simulink model "EX1_PID_pendulum_down"  (R2023b)
settings: Solver=FixedStepDiscrete  StartTime=0.0  StopTime=Inf  FixedStep=Ts  RelTol=1e-3  EnableMultiTasking=on
model workspace (MATLAB code in the model file):
  | % Processor Frequency
  | CPU_frequency = 90e6; %(Hz)
  | 
  | % PWM Settings
  | PWM_frequency = 15e3; %(Hz)
  | PWM_CounterPeriod = CPU_frequency/PWM_frequency/2; %(PWM timer counts)
  | 
  | % Switching frequency
  | fsw = PWM_frequency;
  | 
  | % Integration time (solver)
  | Ts = 1e-4;
  | 
  | % Encoder settings
  | fw = 400; % encoder sampling frequency
  | Tw = 1/fw; % encoder sampling time
values from neighbouring files (symbols this model uses):
  CALIBRATION_TIME = 50    [EX1_init.m]
  K_e = Distance / Encoder_Counts    (= 0.000124665903016)    [EX1_init.m]
  Kd = 0.2    [EX1_init.m]
  Ki = 0    [EX1_init.m]
  Kp = 10    [EX1_init.m]
  x_ref = 0    [EX1_init.m]
undefined symbols (not defined in the file or in its folder): DiscIntNeverNeededParam, Down, GPTRIP1SEL, GPTRIP2SEL, TZ1, TZ2, Up
libraries: c2802xlib x5, dspfdesign x2, simulink x2, c2806xlib x2, dspstat3 x2, c280xlib x1, eeGeneralControl x1, dspsigops x1
settings Model: ExtModeTrigDuration=8  Creator=The MathWorks, Inc.  LastModifiedBy=98912
settings SolverCC: AlgebraicLoopSolver=TrustRegion  AutoInsertRateTranBlk=on
settings OptimizationCC: DefaultUnderspecifiedDataType=single  EnhancedBackFolding=on  PassReuseOutputArgsAs=Individual arguments  MaxStackSize=1024  OptimizeBlockOrder=speed  DifferentSizesBufferReuse=on  OptimizationCustomize=off  DenormalBehavior=FlushToZero  EfficientTunableParamExpr=on
settings DebuggingCC: ParameterTunabilityLossMsg=error  UnconnectedInputMsg=warning  UnconnectedOutputMsg=warning  UnconnectedLineMsg=warning  SubsystemReferenceDiagnosticForUnitTest=warning
settings HardwareCC: ProdBitPerChar=16  ProdBitPerInt=16  ProdBitPerPointer=32  ProdBitPerSizeT=32  ProdBitPerPtrDiffT=32  ProdLargestAtomicInteger=Integer  ProdLargestAtomicFloat=None  ProdWordSize=16  ProdLongLongMode=on  ProdHWDeviceType=Texas Instruments->C2000
settings ModelReferenceCC: EnableRefExpFcnMdlSchedulingChecks=on
settings SFSimCC: MATLABDynamicMemAlloc=off
settings RTWCC: Description=Embedded Coder  SystemTargetFile=ert.tlc  HardwareBoard=TI Piccolo F28069M LaunchPad  TemplateMakefile=ert_default_tmf  GenerateReport=on  Toolchain=Texas Instruments Code Composer Studio (C2000)  DLArmComputeVersion=19.05
settings CodeAppCC: ForceParamTrailComments=on  IgnoreCustomStorageClasses=off  OperatorAnnotations=on  SimulinkDataObjDesc=on  SFDataObjDesc=on  InsertBlockDesc=on
settings ERTTargetCC: CodeReplacementLibrary=TI C28x  ExtModeStaticAllocSize=2000
settings SettingsController: UseSoCProfilerForTargets=0

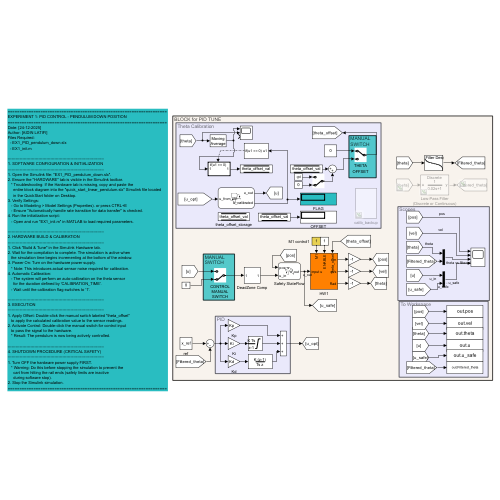
[thumbnail: Simulink's stored preview of the top-level diagram]
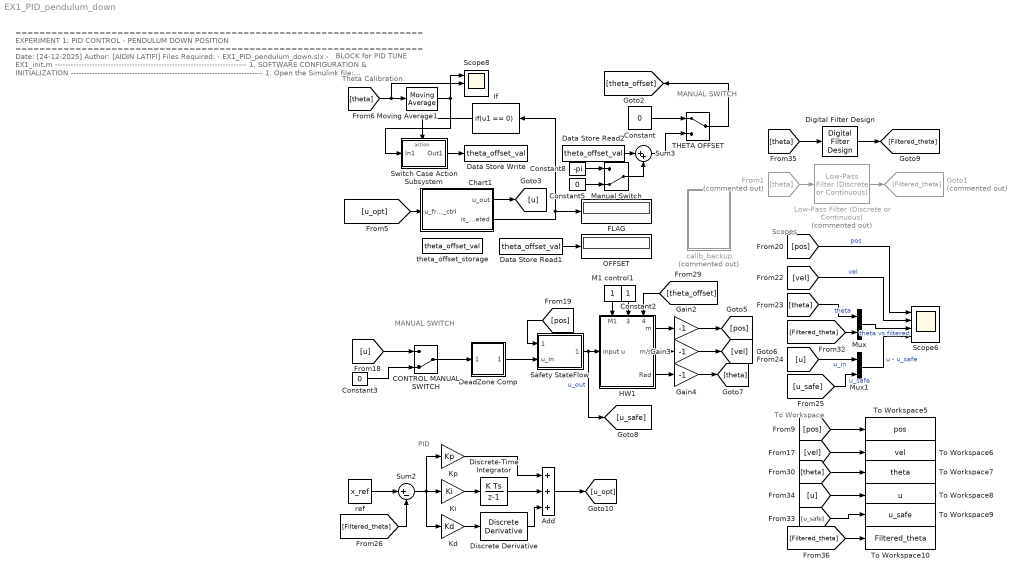
== system EX1_PID_pendulum_down ==
  note: MANUAL
      | SWITCH
  note: ====================================================================
      | EXPERIMENT 1: PID CONTROL - PENDULUM DOWN POSITION
      | ====================================================================
      | Date: [24-12-2025]
      | Author: [AIDIN LATIFI]
      | Files Required:
      |   - EX1_PID_pendulum_down.slx
      |   - EX1_init.m
      |
      | ------------------------------------------------------------------------
      | 1. SOFTWARE CONFIGURATION & INITIALIZATION
      | ------------------------------------------------------------------------
      | 1. Open the Simulink file: "EX1_PID_pendulum_down.slx".
      | 2. Ensure the "HARDWARE" tab is visible in the Simulink toolbar.
      |    * Troubleshooting: If the Hardware tab is missing, copy and paste the
      |      entire block diagram into the "quick_start_linear_pendulum.slx" Simulink file located
      |      in the QuickStart folder on Desktop.
      | 3. Verify Settings:
      |    - Go to Modeling > Model Settings (Properties). or press CTRL+E
      |    - Ensure "Automatically handle rate transition for data transfer" is checked.
      | 4. Run the initialization script:
      |    - Open and run "EX1_init.m" in MATLAB to load required parameters.
      |
      | ------------------------------------------------------------------------
      | 2. HARDWARE BUILD & CALIBRATION
      | ------------------------------------------------------------------------
      | 1. Click "Build & Tune" in the Simulink Hardware tab.
      | 2. Wait for the compilation to complete. The simulation is active when
      |    the simulation time begins incrementing at the bottom of the window.
      | 3. Power On: Turn on the hardware power supply.
      |    * Note: This introduces actual sensor noise required for calibration.
      | 4. Automatic Calibration:
      |    - The system will perform an auto-calibration on the theta sensor
      |      for the duration defined by 'CALIBRATION_TIME'.
      |    - Wait until the calibration flag switches to '1'.
      |
      | ------------------------------------------------------------------------
      | 3. EXECUTION
      | ------------------------------------------------------------------------
      | 1. Apply Offset: Double-click the manual switch labeled "theta_offset"
      |    to apply the calculated calibration value to the sensor readings.
      | 2. Activate Control: Double-click the manual switch for control input
      |    to pass the signal to the hardware.
      |    * Result: The pendulum is now being actively controlled.
      |
      | ------------------------------------------------------------------------
      | 4. SHUTDOWN PROCEDURE (CRITICAL SAFETY)
      | ------------------------------------------------------------------------
      | 1. Turn OFF the hardware power supply FIRST.
      |    * Warning: Do this before stopping the simulation to prevent the
      |      cart from hitting the rail ends (safety limits are inactive
      |      during software stop).
      | 2. Stop the Simulink simulation.
      | ====================================================================
  note: Theta Calibration
  note: To Workspace
  note: BLOCK for PID TUNE
  note: Scopes
  note: PID
  note: MANUAL
      | SWITCH
  Add : Sum  Inputs=+++
  CONTROL MANUAL SWITCH : ManualSwitch  CurrentSetting=0
  Chart1 : Stateflow chart  TreatAsAtomicUnit=on
  Constant : Constant  Value=0  SampleTime=Ts
  Constant2 : Constant
  Constant3 : Constant  Value=0  SampleTime=-1
  Constant5 : Constant  Value=0  SampleTime=Ts
  Constant8 : Constant  Value=-pi  SampleTime=Ts
  Data Store Read1 : DataStoreRead  DataStoreName=theta_offset_val  IndexOptions=Index vector (dialog)  Indices=1  OutputSizes=1
  Data Store Read2 : DataStoreRead  DataStoreName=theta_offset_val  IndexOptions=Index vector (dialog)  Indices=1  OutputSizes=1
  Data Store Write : DataStoreWrite  DataStoreName=theta_offset_val  IndexOptions=Index vector (dialog)  Indices=1  OutputSizes=1
  DeadZone Comp : Subsystem
  Digital Filter Design : dspfdesign/Digital Filter Design  mwdsp_browser_bugfix_var=off
  Discrete Derivative : simulink/Discrete/Discrete Derivative  gainval=1.0  ICPrevScaledInput=0.0  OutMin=[]  OutMax=[]  OutDataType=fixdt(1, 16)  OutScaling=2^-10  DoSatur=off
  Discrete-Time Integrator : DiscreteIntegrator  SampleTime=-1  LimitOutput=on  UpperSaturationLimit=2  LowerSaturationLimit=-2  ICPrevOutput=DiscIntNeverNeededParam  ICPrevScaledInput=DiscIntNeverNeededParam
  FLAG : Display
  From1 : From  Commented=on  GotoTag=theta
  Gain2 : Gain  Gain=-1
  Gain3 : Gain  Gain=-1
  Gain4 : Gain  Gain=-1
  Goto1 : Goto  Commented=on  GotoTag=Filtered_theta
  HW1 : Subsystem
      settings: PortSchema="{\"entries\":[{\"content\":{\"sides\":[{\"content\":{\"connectorIds\":[\"In1\"]},\"type\":\"ConnectorPlacement.EquallySpacedRectSide\",\"uuid\":\"e9898c75-a6e7-4646-b73a-b35b1fbe5adf\"},{\"content\":{\"connectorIds\":[\"Out1\",\"Out2\",\"Out3\"],\"side\":\"RIGHT\"},\"type\":\"ConnectorPlacement.EquallySpacedRectSide\",\"uuid\":\"085d2ccc-0e1f-4b16-8ec9-c70e62f660a1\"},{\"content\":{\"connectorIds\":[\"In2\",\"In3\",\"In4\"],\"side\":\"TOP\"},\"type\":\"ConnectorPlacement.EquallySpacedRectSide\",\"uuid\":\"51882789-74c2-4a7a-a001-ddaf25b9b479\"}]},\"type\":\"ConnectorPlacement.EquallySpacedConnector\",\"uuid\":\"373898fa-4a42-48b4-8ce1-77edd11dc4d5\"}],\"packageUris\":[\"http://schema.mathworks.com/mf0/Connector/R2020b\"],\"version\":\"1.0\"}"
  If : If  IfExpression=u1 == 0  ShowElse=off
  Kd : Gain  Gain=Kd
  Ki : Gain  Gain=Ki
  Kp : Gain  Gain=Kp
  Low-Pass Filter (Discrete or Continuous) : eeGeneralControl/Low-Pass Filter (Discrete or Continuous)  Commented=on  K=1  T=0.02  B=inf  A=-inf  init_option=Inherited from block input  x0=0  Ts=-1
  M1 control1 : Constant
  Manual Switch : ManualSwitch  CurrentSetting=0
  Moving Average1 : dspstat3/Moving Average  Method=Sliding window  ForgettingFactorPort=off  SpecifyWindowLength=off  WindowLength=200  OverlapLength=5  AllowArbitraryInputLength=off  ForgettingFactor=0.9  SimulateUsing=Interpreted execution
  Mux : Mux  Inputs=2
  Mux1 : Mux  Inputs=2
  OFFSET : Display
  Safety StateFlow : Stateflow chart  TreatAsAtomicUnit=on
  Scope6 : Scope  NumInputPorts=4
  Scope8 : Scope  NumInputPorts=3
  Sum2 : Sum  Inputs=|+-
  Sum3 : Sum  Inputs=|++
  Switch Case Action Subsystem : Subsystem  TreatAsAtomicUnit=on
  THETA OFFSET : ManualSwitch
  To Workspace10 : ToWorkspace  VariableName=Filtered_theta  SaveFormat=Timeseries  SampleTime=-1
  To Workspace5 : ToWorkspace  VariableName=pos  SaveFormat=Timeseries  SampleTime=-1
  To Workspace6 : ToWorkspace  VariableName=vel  SaveFormat=Timeseries  SampleTime=-1
  To Workspace7 : ToWorkspace  VariableName=theta  SaveFormat=Timeseries  SampleTime=-1
  To Workspace8 : ToWorkspace  VariableName=u  SaveFormat=Timeseries  SampleTime=-1
  To Workspace9 : ToWorkspace  VariableName=u_safe  SaveFormat=Timeseries  SampleTime=-1
  calib_backup : Subsystem  Commented=on
  ref : Constant  Value=x_ref  SampleTime=-1
  theta_offset_storage : DataStoreMemory  DataStoreName=theta_offset_val  WriteAfterWriteMsg=warning  ShowAdditionalParam=off
  wires:
  [u] -> CONTROL MANUAL SWITCH/1
  [u_safe] -> Mux1/2  "u_safe"
  [vel] -> To Workspace6/1
  Constant/1 -> THETA OFFSET/1
  [pos] -> Scope6/1  "pos"
  Add/1 -> [u_opt]
  Digital Filter Design/1 -> [Filtered_theta]
  [theta_offset] -> HW1/4(Theta_offset)
  Switch Case Action Subsystem/1(Out1) -> Data Store Write/1
  From1/1 -> Low-Pass Filter (Discrete or Continuous)/1
  Safety StateFlow/1(u_out) -> [u_safe], HW1/1(input u)  "u_out"
  Chart1/2(is_calibrated) -> FLAG/1, If/1
  THETA OFFSET/1 -> [theta_offset]
  Ki/1 -> Discrete-Time Integrator/1
  Sum3/1 -> THETA OFFSET/2
  [theta] -> Mux/1  "theta"
  Moving Average1/1 -> Switch Case Action Subsystem/1(In1), Scope8/1
  Data Store Read2/1 -> Sum3/1
  HW1/3(Rad) -> Gain4/1
  Manual Switch/1 -> Sum3/2
  Kd/1 -> Discrete Derivative/1
  Mux1/1 -> Scope6/4  "u - u_safe"
  [theta] -> Scope8/2, Moving Average1/1
  [u_opt] -> Chart1/1(u_from_ctrl)
  Chart1/1(u_out) -> [u]
  Mux/1 -> Scope6/3  "theta vs filtered"
  [Filtered_theta] -> To Workspace10/1
  HW1/2(m/s) -> Gain3/1
  [u] -> Mux1/1  "u_in"
  [pos] -> Safety StateFlow/1(pos_s)
  M1 control1/1 -> HW1/2(M1)
  Constant3/1 -> CONTROL MANUAL SWITCH/2
  Data Store Read1/1 -> OFFSET/1
  If/1 -> Switch Case Action Subsystem/Action
  [Filtered_theta] -> Mux/2
  ref/1 -> Sum2/1
  CONTROL MANUAL SWITCH/1 -> DeadZone Comp/1(In1)
  Constant2/1 -> HW1/3(ENABLE)
  Discrete Derivative/1 -> Add/3
  Constant5/1 -> Manual Switch/2
  Discrete-Time Integrator/1 -> Add/2
  Gain3/1 -> [vel]
  [u] -> To Workspace8/1
  [Filtered_theta] -> Sum2/2
  [pos] -> To Workspace5/1
  Constant8/1 -> Manual Switch/1
  [vel] -> Scope6/2  "vel"
  [theta] -> To Workspace7/1
  Gain4/1 -> [theta]
  [u_safe] -> To Workspace9/1
  DeadZone Comp/1(Out1) -> Safety StateFlow/2(u_in)
  Sum2/1 -> Kd/1, Ki/1, Kp/1
  Gain2/1 -> [pos]
  Kp/1 -> Add/1
  Low-Pass Filter (Discrete or Continuous)/1 -> Goto1/1
  [theta] -> Digital Filter Design/1
  HW1/1(m) -> Gain2/1

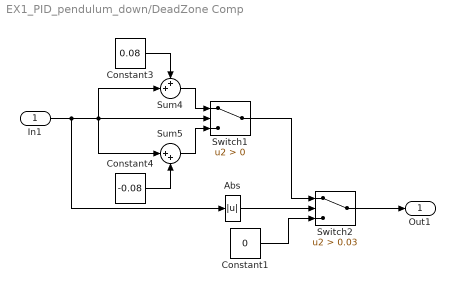
== system EX1_PID_pendulum_down/DeadZone Comp ==
  In1 : Inport
  Abs : Abs  SaturateOnIntegerOverflow=off
  Constant1 : Constant  Value=0  SampleTime=Ts
  Constant3 : Constant  Value=0.08  SampleTime=Ts
  Constant4 : Constant  Value=-0.08  SampleTime=Ts
  Sum4 : Sum  Inputs=++|
  Sum5 : Sum  Inputs=|++
  Switch1 : Switch  Criteria=u2 > Threshold  ZeroCross=off  SaturateOnIntegerOverflow=off  InputSameDT=off
  Switch2 : Switch  Criteria=u2 > Threshold  Threshold=0.03  ZeroCross=off  SaturateOnIntegerOverflow=off  InputSameDT=off
  Out1 : Outport
  wires:
  Switch2/1 -> Out1/1
  Constant1/1 -> Switch2/3
  Abs/1 -> Switch2/2
  In1/1 -> Abs/1, Switch1/2, Sum4/2, Sum5/1
  Constant4/1 -> Sum5/2
  Sum4/1 -> Switch1/1
  Switch1/1 -> Switch2/1
  Sum5/1 -> Switch1/3
  Constant3/1 -> Sum4/1

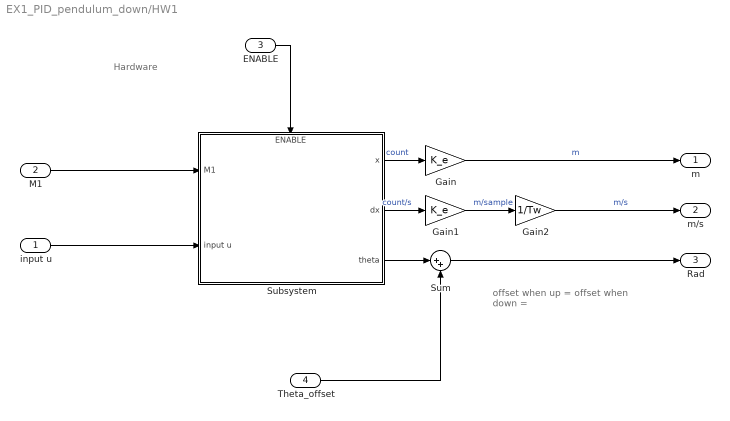
== system EX1_PID_pendulum_down/HW1 ==
  note: Hardware
  note: offset when up =
      | offset when down =
  input u : Inport
  M1 : Inport  Port=2
  ENABLE : Inport  Port=3
  Theta_offset : Inport  Port=4
  Gain : Gain  Gain=K_e
  Gain1 : Gain  Gain=K_e
  Gain2 : Gain  Gain=1/Tw
  Subsystem : Subsystem
      settings: PortSchema="{\"entries\":[{\"content\":{\"sides\":[{\"content\":{\"connectorIds\":[\"In1\",\"In2\"]},\"type\":\"ConnectorPlacement.EquallySpacedRectSide\",\"uuid\":\"8c9bf6c9-d924-4f96-91b5-abbbae04c6cc\"},{\"content\":{\"connectorIds\":[\"Out1\",\"Out2\",\"Out3\"],\"side\":\"RIGHT\"},\"type\":\"ConnectorPlacement.EquallySpacedRectSide\",\"uuid\":\"103da16e-06eb-4691-82c0-4f59d0e2dd5c\"},{\"content\":{\"connectorIds\":[\"In3\"],\"side\":\"TOP\"},\"type\":\"ConnectorPlacement.EquallySpacedRectSide\",\"uuid\":\"54cad98e-2bed-4b56-a022-16556b8a0715\"}]},\"type\":\"ConnectorPlacement.EquallySpacedConnector\",\"uuid\":\"c42b460b-a194-4c24-b642-2d9f844fa4d6\"}],\"packageUris\":[\"http://schema.mathworks.com/mf0/Connector/R2020b\"],\"version\":\"1.0\"}"
  Sum : Sum  Inputs=|++
  m : Outport
  m/s : Outport  Port=2
  Rad : Outport  Port=3
  wires:
  ENABLE/1 -> Subsystem/3(ENABLE)
  Sum/1 -> Rad/1
  M1/1 -> Subsystem/1(M1)
  Subsystem/3(theta) -> Sum/1
  Subsystem/2(dx) -> Gain1/1  "count/s"
  Subsystem/1(x) -> Gain/1  "count"
  Gain1/1 -> Gain2/1  "m/sample"
  input u/1 -> Subsystem/2(input u)
  Theta_offset/1 -> Sum/2
  Gain/1 -> m/1  "m"
  Gain2/1 -> m/s/1  "m/s"

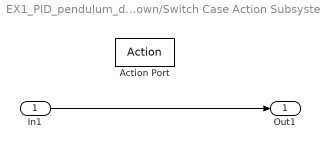
== system EX1_PID_pendulum_down/Switch Case Action Subsystem ==
  In1 : Inport
  Action Port : ActionPort  ActionPortLabel=if(u1 == 0)
  Out1 : Outport
  wires:
  In1/1 -> Out1/1

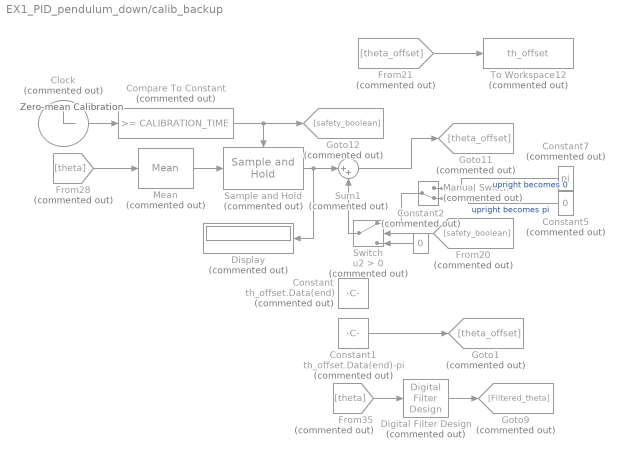
== system EX1_PID_pendulum_down/calib_backup ==
  note: Zero-mean Calibration
  Clock : Clock  Commented=on
  Compare To Constant : simulink/Logic and Bit Operations/Compare To Constant  Commented=on  relop=>=  const=CALIBRATION_TIME  OutDataTypeStr=boolean
  Constant : Constant  Commented=on  Value=th_offset.Data(end)
  Constant1 : Constant  Commented=on  Value=th_offset.Data(end)-pi
  Constant2 : Constant  Commented=on  Value=0  SampleTime=-1
  Constant5 : Constant  Commented=on  Value=0  SampleTime=-1
  Constant7 : Constant  Commented=on  Value=pi  SampleTime=-1
  Digital Filter Design : dspfdesign/Digital Filter Design  Commented=on  mwdsp_browser_bugfix_var=off
  Display : Display  Commented=on
  From20 : From  Commented=on  GotoTag=safety_boolean
  From21 : From  Commented=on  GotoTag=theta_offset
  From28 : From  Commented=on  GotoTag=theta
  From35 : From  Commented=on  GotoTag=theta
  Goto1 : Goto  Commented=on  GotoTag=theta_offset
  Goto11 : Goto  Commented=on  GotoTag=theta_offset
  Goto12 : Goto  Commented=on  GotoTag=safety_boolean
  Goto9 : Goto  Commented=on  GotoTag=Filtered_theta
  Manual Switch4 : ManualSwitch  Commented=on  CurrentSetting=0
  Mean : dspstat3/Mean  Commented=on  run=off  InputProcessing=Columns as channels (frame based)  reset_popup=None  directionMode=Each column  dimension=1  roiEnable=off  roiType=Rectangles  roiPortion=Entire ROI  roiOutput=Individual statistics for each ROI  roiFlag=off  roundingMode=Floor  overflowMode=off  outputDataTypeStr=Inherit: Same as accumulator  outputMin=[]  outputMax=[]  outputLastDataTypeStr=Inherit: Same as accumulator
  Sample and Hold : dspsigops/Sample and Hold  Commented=on  trig=Rising edge  initCond=0  latchinput=on
  Sum1 : Sum  Commented=on  Inputs=|++
  Switch : Switch  Commented=on  Criteria=u2 > Threshold  SaturateOnIntegerOverflow=off  InputSameDT=off
  To Workspace12 : ToWorkspace  Commented=on  VariableName=th_offset  SaveFormat=Timeseries  SampleTime=-1
  wires:
  Constant1/1 -> Goto1/1
  Compare To Constant/1 -> Sample and Hold/Trigger, Goto12/1
  Digital Filter Design/1 -> Goto9/1
  Sum1/1 -> Goto11/1
  Sample and Hold/1 -> Display/1, Sum1/1
  From28/1 -> Mean/1
  Switch/1 -> Sum1/2
  Mean/1 -> Sample and Hold/1
  From35/1 -> Digital Filter Design/1
  From21/1 -> To Workspace12/1
  Constant2/1 -> Switch/3
  Constant7/1 -> Manual Switch4/1  "upright becomes 0"
  Clock/1 -> Compare To Constant/1
  Constant5/1 -> Manual Switch4/2  "upright becomes pi"
  From20/1 -> Switch/2
  Manual Switch4/1 -> Switch/1

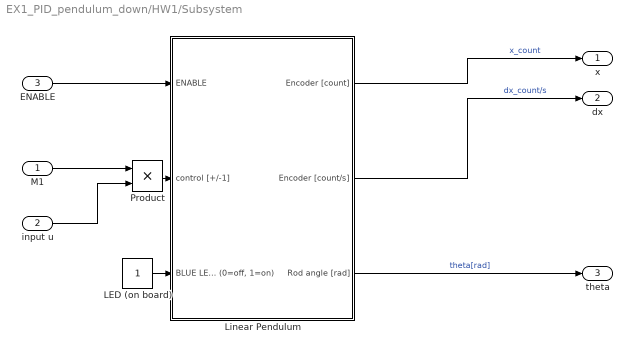
== system EX1_PID_pendulum_down/HW1/Subsystem ==
  M1 : Inport
  input u : Inport  Port=2
  ENABLE : Inport  Port=3
  LED (on board) : Constant  SampleTime=0.5
  Linear Pendulum : Subsystem
  Product : Product
  x : Outport
  dx : Outport  Port=2
  theta : Outport  Port=3
  wires:
  ENABLE/1 -> Linear Pendulum/1(ENABLE)
  Linear Pendulum/1(Encoder [count]) -> x/1  "x_count"
  LED (on board)/1 -> Linear Pendulum/3("BLUE LED (0=off, 1=on)")
  Product/1 -> Linear Pendulum/2(control [+/-1])
  Linear Pendulum/3(Rod angle [rad]) -> theta/1  "theta[rad]"
  input u/1 -> Product/2
  Linear Pendulum/2(Encoder [count/s]) -> dx/1  "dx_count/s"
  M1/1 -> Product/1

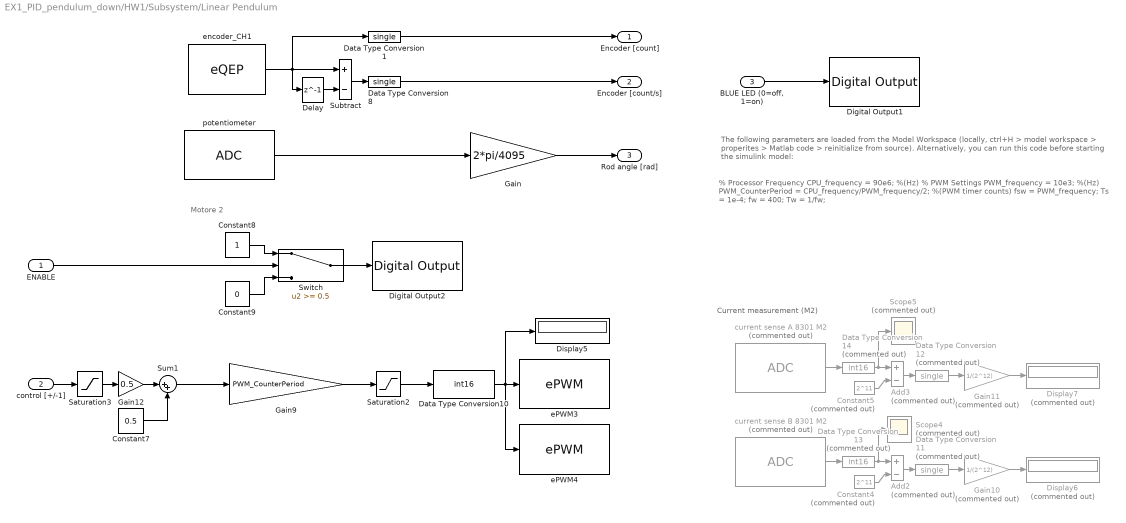
== system EX1_PID_pendulum_down/HW1/Subsystem/Linear Pendulum ==
  note: Current measurement (M2)
  note: The following parameters are loaded from the Model Workspace (locally, ctrl+H > model workspace > properites > Matlab code > reinitialize from source). Alternatively, you can run this code before starting the simulink model:
  note: % Processor Frequency
      | CPU_frequency = 90e6; %(Hz)
      | % PWM Settings
      | PWM_frequency = 10e3; %(Hz)
      | PWM_CounterPeriod = CPU_frequency/PWM_frequency/2; %(PWM timer counts)
      | fsw = PWM_frequency;
      | Ts = 1e-4;
      | fw = 400;
      | Tw = 1/fw;
  note: Motore 2
  ENABLE : Inport
  control [+/-1] : Inport  Port=2
  "BLUE LED (0=off, 1=on)" : Inport  Port=3
  Add2 : Sum  Commented=on  Inputs=+-
  Add3 : Sum  Commented=on  Inputs=+-
  Constant4 : Constant  Commented=on  Value=2^11  OutDataTypeStr=int16  SampleTime=Ts*10
  Constant5 : Constant  Commented=on  Value=2^11  OutDataTypeStr=int16  SampleTime=Ts*10
  Constant7 : Constant  Value=0.5
  Constant8 : Constant
  Constant9 : Constant  Value=0
  Data Type Conversion1 : DataTypeConversion  OutDataTypeStr=single  SaturateOnIntegerOverflow=off  RndMeth=Floor
  Data Type Conversion10 : DataTypeConversion  OutDataTypeStr=int16  SaturateOnIntegerOverflow=off  RndMeth=Floor
  Data Type Conversion11 : DataTypeConversion  Commented=on  OutDataTypeStr=single  SaturateOnIntegerOverflow=off  RndMeth=Floor
  Data Type Conversion12 : DataTypeConversion  Commented=on  OutDataTypeStr=single  SaturateOnIntegerOverflow=off  RndMeth=Floor
  Data Type Conversion13 : DataTypeConversion  Commented=on  OutDataTypeStr=int16  SaturateOnIntegerOverflow=off  RndMeth=Floor
  Data Type Conversion14 : DataTypeConversion  Commented=on  OutDataTypeStr=int16  SaturateOnIntegerOverflow=off  RndMeth=Floor
  Data Type Conversion8 : DataTypeConversion  OutDataTypeStr=single  SaturateOnIntegerOverflow=off  RndMeth=Floor
  Delay : Delay  DelayLength=1  SampleTime=Tw
  Digital Output1 : c2806xlib/Digital Output  GPIO_Number=GPIO32~GPIO39  GPIO_Bit0=off  GPIO_BIT0_Toggle=off  GPIO_Bit1=off  GPIO_BIT1_Toggle=off  GPIO_Bit2=off  GPIO_BIT2_Toggle=off  GPIO_Bit3=off  GPIO_BIT3_Toggle=off  GPIO_Bit4=off  GPIO_BIT4_Toggle=off  GPIO_Bit5=off  GPIO_BIT5_Toggle=off  GPIO_Bit6=off  GPIO_BIT6_Toggle=off  GPIO_Bit7=on  GPIO_BIT7_Toggle=on
  Digital Output2 : c2806xlib/Digital Output  GPIO_Number=GPIO8~GPIO15  GPIO_Bit0=off  GPIO_BIT0_Toggle=off  GPIO_Bit1=off  GPIO_BIT1_Toggle=off  GPIO_Bit2=off  GPIO_BIT2_Toggle=off  GPIO_Bit3=off  GPIO_BIT3_Toggle=off  GPIO_Bit4=on  GPIO_BIT4_Toggle=off  GPIO_Bit5=off  GPIO_BIT5_Toggle=off  GPIO_Bit6=off  GPIO_BIT6_Toggle=off  GPIO_Bit7=off  GPIO_BIT7_Toggle=off
  Display5 : Display
  Display6 : Display  Commented=on
  Display7 : Display  Commented=on
  Gain : Gain  Gain=2*pi/4095
  Gain10 : Gain  Commented=on  Gain=1/(2^12)
  Gain11 : Gain  Commented=on  Gain=1/(2^12)
  Gain12 : Gain  Gain=0.5
  Gain9 : Gain  Gain=PWM_CounterPeriod
  Saturation2 : Saturate  UpperLimit=PWM_CounterPeriod  LowerLimit=0
  Saturation3 : Saturate  UpperLimit=1  LowerLimit=-1
  Scope4 : Scope  Commented=on
  Scope5 : Scope  Commented=on
  Subtract : Sum  Inputs=+-
  Sum1 : Sum  Inputs=|++
  Switch : Switch  Threshold=0.5  SaturateOnIntegerOverflow=off  InputSameDT=off
  current sense A 8301 M2 : c2802xlib/ADC  Commented=on  blkParamProc=C2000  ADCModule=1  samplingMode=Single sample mode  ADCResolution=12-bit (Single-ended input)  useSOC1=SOC3  useSOC2=SOC0_SOC1  SOCAcquisitionWindow=7  SOCTriggerSource=ePWM4_ADCSOCA  SOCInterruptTrigger=No ADCINT  Ts=Ts*10  dType=uint16  postInterrupt=off  interruptSel=ADCINT1  ADCINTContinuous=on  endma=off  chdma=1  conv1=ADCINA3  conv2=ADCINA0 and ADCINB0  conv1_Type4=ADCIN0  conv2_Type4=ADCIN0 and ADCIN1
  current sense B 8301 M2 : c2802xlib/ADC  Commented=on  blkParamProc=C2000  ADCModule=1  samplingMode=Single sample mode  ADCResolution=12-bit (Single-ended input)  useSOC1=SOC4  useSOC2=SOC0_SOC1  SOCAcquisitionWindow=7  SOCTriggerSource=ePWM5_ADCSOCA  SOCInterruptTrigger=No ADCINT  Ts=Ts*10  dType=uint16  postInterrupt=off  interruptSel=ADCINT1  ADCINTContinuous=on  endma=off  chdma=1  conv1=ADCINB3  conv2=ADCINA0 and ADCINB0  conv1_Type4=ADCIN0  conv2_Type4=ADCIN0 and ADCIN1
  ePWM3 : c2802xlib/ePWM  PwmType=C2000  useModule=ePWM1  ePWMxLINKTBPRD=Not Linked  periodUnits=Clock cycles  timerSource=Specify via dialog  timerPeriod_clk=PWM_CounterPeriod+1  timerPeriod_sec=0.0001  tbshadow=Counter equals to zero  countingMode=Up-Down  phaseActiveEnable=Disable  phaseDirection=Count down after sync  phaseActive=0  synchronizationEnable=off  dcaevt1Sync=off  dcbevt1Sync=off  synchronizationOption=Disable  dcbevt1SyncOut=off  dcaevt1SyncOut=off  cmpdSyncOut=off  cmpcSyncOut=off  cmpbSyncOut=off  zeroSyncOut=off  swfSyncOut=off  perSynchronizationOption=Counter equals to period (CTR=PRD)  clockPrescale=1  HSclockPrescale=1  enswap=off  ePWMxAStatus=on  ePWMxAactionLogic1=Do nothing  ePWMxAactionLogic2=Do nothing  ePWMxAactionLogic3=Clear  ePWMxAactionLogic4=Set  ePWMxAactionLogic5=Do nothing  ePWMxAactionLogic6=Do nothing  ePWMxACSFenable=off  ePWMxACSFvalue=Forcing disable  ePWMxASFreload=Zero  ePWMxBStatus=off  ePWMxBactionLogic1=Set  ePWMxBactionLogic2=Clear  ePWMxBactionLogic3=Do nothing  ePWMxBactionLogic4=Do nothing  ePWMxBactionLogic5=Clear  ePWMxBactionLogic6=Set  ePWMxBCSFenable=off  ePWMxBCSFvalue=Forcing disable  ePWMxBSFreload=Zero  ePWNxBOutWay=on  ePWMxLINKCMPA=Not Linked  CMPAUnits=Clock cycles  CMPASource=Input port  CMPAValue_per=50  CMPAValue_clk=PWM_CounterPeriod/2+1  enCMPAshadow=Counter equals to zero (CTR=Zero)  ePWMxLINKCMPB=Not Linked  CMPBUnits=Clock cycles  CMPBSource=Specify via dialog  CMPBValue_per=50  CMPBValue_clk=PWM_CounterPeriod/2 +1  enCMPBshadow=Counter equals to zero (CTR=Zero)  ePWMxLINKCMPC=Not Linked  CMPCUnits=Clock cycles  CMPCSource=Specify via dialog  CMPCValue_per=50  CMPCValue_clk=32000  enCMPCshadow=Counter equals to zero (CTR=Zero)  ePWMxLINKCMPD=Not Linked  CMPDUnits=Clock cycles  CMPDSource=Specify via dialog  CMPDValue_per=50  CMPDValue_clk=32000  enCMPDshadow=Counter equals to zero (CTR=Zero)  enableDBePWMxA=on  enableDBePWMxB=on  enhalfcycle=off  DBpolarity=Active high (AH)  DBedgeDelay=Positive  DBSource_ePWMxA=ePWMxA  DBSource_ePWMxB=ePWMxA  DBPeriodUnits=Clock cycles  DBperiodSource=Specify via dialog  REDperiod=15  FEDperiod=15  REDperiod_sec=0  FEDperiod_sec=0  LoadModeDBRED=Immediate without using shadow  LoadModeDBFED=Immediate without using shadow  adcstartModuleA=on  adcrequestEventA=First event  adcstartEventA=Counter equals to period (CTR=PRD)  adcstartEventA_type2=Digital Compare Module A Event 1 start of conversion (DCAEVT1.soc)  adcstartModuleB=off  adcrequestEventB=First event  adcstartEventB=Counter equals to zero (CTR=Zero)  adcstartEventB_type2=Counter equals to zero (CTR=Zero)  intEn=off  intPrd=First event  intSel=Counter equals to zero (CTR=Zero)  intSel_type2=Counter equals to zero (CTR=Zero)  hrpe=off  enHRPWM=off  HRPWM_LoadMode=Counter equals to period (CTR=PRD)  HRPWM_CTLMode=Duty or Period control mode  HRPWM_EDGMode=Both edge  hrpeb=off  enHRPWMB=off  HRPWM_LoadModeB=Counter equals to zero (CTR=ZERO)  HRPWM_CTLModeB=Duty or Period control mode  HRPWM_EDGModeB=Both edge  enHRDBRED=off  enHRDBFED=off  enSFO=on  enautoconv=on  chopperEnable=off  chopperFrequency=1  chopperFirstwidth=1  chopperDuty=12.5%  tripZonesource=Specify via dialog  tzselOSHT1=off  tzselOSHT2=off  tzselOSHT3=off  tzselOSHT4=off  tzselOSHT5=off  tzselOSHT6=off  tzselOSHDCAEV1=off  tzselOSHDCBEV1=off  tzselCBC1=off  tzselCBC2=off  tzselCBC3=off  tzselCBC4=off  tzselCBC5=off  tzselCBC6=off  tzselCBCDCAEV2=off  tzselCBCDCBEV2=off  enTzOstIntr=off  enTzCbcIntr=off  enTzDCAEVT1Intr=off  enTzDCAEVT2Intr=off  enTzDCBEVT1Intr=off  enTzDCBEVT2Intr=off  tzclrCBCLatch=Counter equals to zero (CTR=Zero)  ePWMxAforced=No action  ePWMxBforced=No action  DCAEVT1forced=No action  DCBEVT1forced=No action  DCAEVT2forced=No action  DCBEVT2forced=No action  dcah=Trip Zone 1 input (TZ1)  dcal=Trip Zone 2 input (TZ2)  dcbh=Trip Zone 1 input (TZ1)  dcbl=Trip Zone 2 input (TZ2)  dcah_type2=GPTRIP1SEL/(TZ1)  dcal_type2=GPTRIP2SEL/(TZ2)  dcbh_type2=GPTRIP1SEL/(TZ1)  dcbl_type2=GPTRIP2SEL/(TZ2)  gendcaevt1=Event disabled  gendcaevt2=Event disabled  gendcbevt1=Event disabled  gendcbevt2=Event disabled  dcaevt1src=DCAEVT1 with sync  dcaevt2src=DCAEVT2 with sync  dcbevt1src=DCBEVT1 with sync  dcbevt2src=DCBEVT2 with sync  pulsesel=Counter equals to zero (CTR=Zero)  blankinv=off  blankoffset=0  blankwidth=0  evsrcsel=Filtered version of DCAEVT1 (DCAEVT1FILT)  encape=off
  ePWM4 : c2802xlib/ePWM  PwmType=C2000  useModule=ePWM2  ePWMxLINKTBPRD=Not Linked  periodUnits=Clock cycles  timerSource=Specify via dialog  timerPeriod_clk=PWM_CounterPeriod+1  timerPeriod_sec=0.0001  tbshadow=Counter equals to zero  countingMode=Up-Down  phaseActiveEnable=Disable  phaseDirection=Count down after sync  phaseActive=0  synchronizationEnable=off  dcaevt1Sync=off  dcbevt1Sync=off  synchronizationOption=Disable  dcbevt1SyncOut=off  dcaevt1SyncOut=off  cmpdSyncOut=off  cmpcSyncOut=off  cmpbSyncOut=off  zeroSyncOut=off  swfSyncOut=off  perSynchronizationOption=Counter equals to period (CTR=PRD)  clockPrescale=1  HSclockPrescale=1  enswap=on  ePWMxAStatus=on  ePWMxAactionLogic1=Do nothing  ePWMxAactionLogic2=Do nothing  ePWMxAactionLogic3=Clear  ePWMxAactionLogic4=Set  ePWMxAactionLogic5=Do nothing  ePWMxAactionLogic6=Do nothing  ePWMxACSFenable=off  ePWMxACSFvalue=Forcing disable  ePWMxASFreload=Zero  ePWMxBStatus=off  ePWMxBactionLogic1=Set  ePWMxBactionLogic2=Clear  ePWMxBactionLogic3=Do nothing  ePWMxBactionLogic4=Do nothing  ePWMxBactionLogic5=Clear  ePWMxBactionLogic6=Set  ePWMxBCSFenable=off  ePWMxBCSFvalue=Forcing disable  ePWMxBSFreload=Zero  ePWNxBOutWay=on  ePWMxLINKCMPA=Not Linked  CMPAUnits=Clock cycles  CMPASource=Input port  CMPAValue_per=50  CMPAValue_clk=PWM_CounterPeriod/2+1  enCMPAshadow=Counter equals to zero (CTR=Zero)  ePWMxLINKCMPB=Not Linked  CMPBUnits=Clock cycles  CMPBSource=Specify via dialog  CMPBValue_per=50  CMPBValue_clk=PWM_CounterPeriod/2 +1  enCMPBshadow=Counter equals to zero (CTR=Zero)  ePWMxLINKCMPC=Not Linked  CMPCUnits=Clock cycles  CMPCSource=Specify via dialog  CMPCValue_per=50  CMPCValue_clk=32000  enCMPCshadow=Counter equals to zero (CTR=Zero)  ePWMxLINKCMPD=Not Linked  CMPDUnits=Clock cycles  CMPDSource=Specify via dialog  CMPDValue_per=50  CMPDValue_clk=32000  enCMPDshadow=Counter equals to zero (CTR=Zero)  enableDBePWMxA=on  enableDBePWMxB=on  enhalfcycle=off  DBpolarity=Active high (AH)  DBedgeDelay=Positive  DBSource_ePWMxA=ePWMxA  DBSource_ePWMxB=ePWMxA  DBPeriodUnits=Clock cycles  DBperiodSource=Specify via dialog  REDperiod=15  FEDperiod=15  REDperiod_sec=0  FEDperiod_sec=0  LoadModeDBRED=Immediate without using shadow  LoadModeDBFED=Immediate without using shadow  adcstartModuleA=on  adcrequestEventA=First event  adcstartEventA=Counter equals to period (CTR=PRD)  adcstartEventA_type2=Digital Compare Module A Event 1 start of conversion (DCAEVT1.soc)  adcstartModuleB=off  adcrequestEventB=First event  adcstartEventB=Counter equals to zero (CTR=Zero)  adcstartEventB_type2=Counter equals to zero (CTR=Zero)  intEn=off  intPrd=First event  intSel=Counter equals to zero (CTR=Zero)  intSel_type2=Counter equals to zero (CTR=Zero)  hrpe=off  enHRPWM=off  HRPWM_LoadMode=Counter equals to period (CTR=PRD)  HRPWM_CTLMode=Duty or Period control mode  HRPWM_EDGMode=Both edge  hrpeb=off  enHRPWMB=off  HRPWM_LoadModeB=Counter equals to zero (CTR=ZERO)  HRPWM_CTLModeB=Duty or Period control mode  HRPWM_EDGModeB=Both edge  enHRDBRED=off  enHRDBFED=off  enSFO=on  enautoconv=on  chopperEnable=off  chopperFrequency=1  chopperFirstwidth=1  chopperDuty=12.5%  tripZonesource=Specify via dialog  tzselOSHT1=off  tzselOSHT2=off  tzselOSHT3=off  tzselOSHT4=off  tzselOSHT5=off  tzselOSHT6=off  tzselOSHDCAEV1=off  tzselOSHDCBEV1=off  tzselCBC1=off  tzselCBC2=off  tzselCBC3=off  tzselCBC4=off  tzselCBC5=off  tzselCBC6=off  tzselCBCDCAEV2=off  tzselCBCDCBEV2=off  enTzOstIntr=off  enTzCbcIntr=off  enTzDCAEVT1Intr=off  enTzDCAEVT2Intr=off  enTzDCBEVT1Intr=off  enTzDCBEVT2Intr=off  tzclrCBCLatch=Counter equals to zero (CTR=Zero)  ePWMxAforced=No action  ePWMxBforced=No action  DCAEVT1forced=No action  DCBEVT1forced=No action  DCAEVT2forced=No action  DCBEVT2forced=No action  dcah=Trip Zone 1 input (TZ1)  dcal=Trip Zone 2 input (TZ2)  dcbh=Trip Zone 1 input (TZ1)  dcbl=Trip Zone 2 input (TZ2)  dcah_type2=GPTRIP1SEL/(TZ1)  dcal_type2=GPTRIP2SEL/(TZ2)  dcbh_type2=GPTRIP1SEL/(TZ1)  dcbl_type2=GPTRIP2SEL/(TZ2)  gendcaevt1=Event disabled  gendcaevt2=Event disabled  gendcbevt1=Event disabled  gendcbevt2=Event disabled  dcaevt1src=DCAEVT1 with sync  dcaevt2src=DCAEVT2 with sync  dcbevt1src=DCBEVT1 with sync  dcbevt2src=DCBEVT2 with sync  pulsesel=Counter equals to zero (CTR=Zero)  blankinv=off  blankoffset=0  blankwidth=0  evsrcsel=Filtered version of DCAEVT1 (DCAEVT1FILT)  encape=off
  encoder_CH1 : c280xlib/eQEP  useModule=eQEP1  pcInputmode=Quadrature-count  externalClockrate=2x resolution: Count the rising/falling edge  swapPolarityselection=Clockwise  qdfOutputport=off  qapPolarityselection=off  qbpPolarityselection=off  qipPolarityselection=off  qspPolarityselection=off  igatePolarityselection=off  sampleTime=Tw  pcOutputport=on  pcMaximumvalue=4294967295  indexInitializationcheck=off  indexInitializationevent=Rising edge  strobeInitializationcheck=off  strobeInitializationevent=Rising edge  softwareInitializationcheck=on  softwareInitializationsource=Set to init value at start up  softwareInitializationmode=on  pcInitialvalue=0  pcResetmode=Reset on the maximum position  ieloutputport=off  indexEventlatch=Rising edge  seloutputport=off  strobeEventlatch=Rising edge  pcefOutputport=off  enableEqepcapture=off  qctmrOutputport=off  qcprdOutputport=off  captureTimerprescaler=1  upEventprescaler=1  overflowErrorflag=off  directionErrorflag=off  captureTimerposition=On unit time-out event  unitTimerperiod=100000000*0+4294967295  captureTimerlatch=off  capturePeriodlatch=off  positionCounterlatch=on  soenPolarityselection=off  spselPolarityselection=Index pin is used for sync output  compareValuesource=Specify via dialog  shadowMode=Load on QPOSCNT=0  compareValue=4294967295  syncOutputwidth=1  polaritySyncoutput=Active high  watchdogEnable=off  watchdogTimer=65535  outport1Datatype=auto  outport2Datatype=int32  outport3Datatype=auto  outport4Datatype=auto  outport5Datatype=auto  outport6Datatype=uint32  outport7Datatype=uint32  outport8Datatype=auto  outport9Datatype=auto  outport10Datatype=auto  outport11Datatype=auto  outport12Datatype=auto  eqepinterrupt_pce=off  eqepinterrupt_qpe=off  eqepinterrupt_qdc=off  eqepinterrupt_wto=off  eqepinterrupt_pcu=off  eqepinterrupt_pco=off  eqepinterrupt_pcr=off  eqepinterrupt_pcm=off  eqepinterrupt_sel=off  eqepinterrupt_iel=off  eqepinterrupt_uto=off  pheOutputport=off  watchdogOutputport=off  outport13Datatype=auto  outport14Datatype=auto
  potentiometer : c2802xlib/ADC  blkParamProc=C2000  ADCModule=1  samplingMode=Single sample mode  ADCResolution=12-bit (Single-ended input)  useSOC1=SOC4  useSOC2=SOC0_SOC1  SOCAcquisitionWindow=7  SOCTriggerSource=CPU0_TINT0n  SOCInterruptTrigger=No ADCINT  Ts=Ts*10  dType=single  postInterrupt=off  interruptSel=ADCINT1  ADCINTContinuous=on  endma=off  chdma=1  conv1=ADCINB7  conv2=ADCINA0 and ADCINB0  conv1_Type4=ADCIN0  conv2_Type4=ADCIN0 and ADCIN1
  Encoder [count] : Outport
  Encoder [count/s] : Outport  Port=2
  Rod angle [rad] : Outport  Port=3
  wires:
  Constant4/1 -> Add2/2
  Add3/1 -> Data Type Conversion12/1
  Data Type Conversion14/1 -> Add3/1, Scope5/1
  Saturation2/1 -> Data Type Conversion10/1
  Data Type Conversion13/1 -> Add2/1, Scope4/1
  Data Type Conversion10/1 -> ePWM4/1, Display5/1, ePWM3/1
  current sense A 8301 M2/1 -> Data Type Conversion14/1
  Data Type Conversion11/1 -> Gain10/1
  Data Type Conversion12/1 -> Gain11/1
  Gain10/1 -> Display6/1
  Gain11/1 -> Display7/1
  Delay/1 -> Subtract/2
  Add2/1 -> Data Type Conversion11/1
  Constant5/1 -> Add3/2
  current sense B 8301 M2/1 -> Data Type Conversion13/1
  Gain9/1 -> Saturation2/1
  encoder_CH1/1 -> Data Type Conversion1/1, Subtract/1, Delay/1
  Subtract/1 -> Data Type Conversion8/1
  "BLUE LED (0=off, 1=on)"/1 -> Digital Output1/1
  Constant7/1 -> Sum1/2
  Gain12/1 -> Sum1/1
  Sum1/1 -> Gain9/1
  Switch/1 -> Digital Output2/1
  ENABLE/1 -> Switch/2
  Constant8/1 -> Switch/1
  Constant9/1 -> Switch/3
  Saturation3/1 -> Gain12/1
  control [+/-1]/1 -> Saturation3/1
  Data Type Conversion8/1 -> Encoder [count/s]/1
  Data Type Conversion1/1 -> Encoder [count]/1
  potentiometer/1 -> Gain/1
  Gain/1 -> Rod angle [rad]/1

== stateflow chart EX1_PID_pendulum_down/Safety StateFlow ==
  state RecoverFrom_UpperBound
    state Halt
      entry: u_out = 0;
    state HomingPulse
      entry:
      u_out = -0.2;
    state PostHomingWait
      entry:
      u_out = 0;
    state wait
      entry:
      flag = 1;
    (default) -> RecoverFrom_UpperBound.Halt
    RecoverFrom_UpperBound.Halt -> RecoverFrom_UpperBound.HomingPulse : [after(3,sec)]
    RecoverFrom_UpperBound.PostHomingWait -> RecoverFrom_UpperBound.wait : [after(3,sec)]
    RecoverFrom_UpperBound.HomingPulse -> RecoverFrom_UpperBound.PostHomingWait : [after(PULSE_TIME,sec)]
  state NormalOpertaion
    u_out = u_in;
    flag=0;
  state RecoverFrom_LowerBound
    state Halt
      entry: u_out = 0;
    state HomingPulse
      entry:
      u_out = 0.2;
    state PostHomingWait
      entry:
      u_out = 0;
    state wait
      entry:
      flag = 1;
    (default) -> RecoverFrom_LowerBound.Halt
    RecoverFrom_LowerBound.Halt -> RecoverFrom_LowerBound.HomingPulse : [[after(3,sec)]]
    RecoverFrom_LowerBound.HomingPulse -> RecoverFrom_LowerBound.PostHomingWait : [[after(PULSE_TIME,sec)]]
    RecoverFrom_LowerBound.PostHomingWait -> RecoverFrom_LowerBound.wait : [[after(3,sec)]]
  RecoverFrom_UpperBound -> NormalOpertaion : [flag==1]
  NormalOpertaion -> RecoverFrom_UpperBound [order 1] : [pos_s>0.25]
  (default) -> NormalOpertaion
  RecoverFrom_LowerBound -> NormalOpertaion : [[flag==1]]
  NormalOpertaion -> RecoverFrom_LowerBound [order 2] : [pos_s<-0.25]
  data: pos_s input; u_in input; PULSE_TIME constant double =1.8; u_out output; flag local =0

== stateflow chart EX1_PID_pendulum_down/Chart1 ==
  state Calibrating
    entry:
    u_out = 0;
    is_calibrated = 0;
  state Controlling
    entry:
    is_calibrated = 1;
    during:
    u_out = u_from_ctrl;
  (default) -> Calibrating
  Calibrating -> Controlling : after(CALIBRATION_TIME, sec)
  data: u_from_ctrl input; u_out output; is_calibrated output; CALIBRATION_TIME constant double =50
